simulink model "MEEN432_Project3_Wk3_Model"  (R2024b)
settings: Solver=VariableStepAuto  StartTime=0.0  StopTime=344  RelTol=1e-3
values from neighbouring files (symbols this model uses):
  epa = urban_epa    [Project3_run.m]
  time = urban_time    [Project3_run.m]
undefined symbols (not defined in the file or in its folder): datBat, datCar, datMotor, F_drag, I_w, m, r
libraries: slpidlib x2
settings Model: Creator=flare  LastModifiedBy=jpalm
settings RTWCC: GPUComputeCapability=3.5

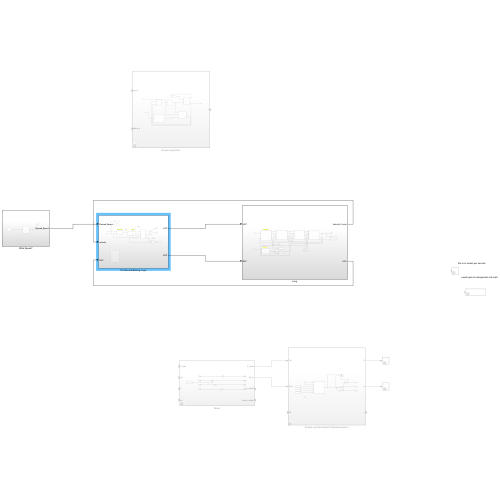
[thumbnail: Simulink's stored preview of the top-level diagram]
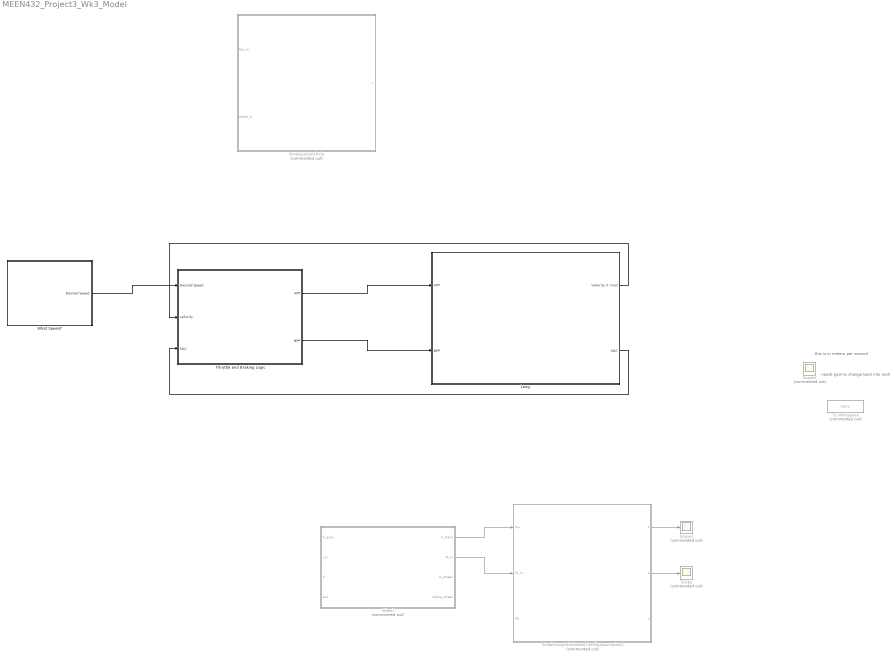
== system MEEN432_Project3_Wk3_Model ==
  note: needs gain to change back into mph
  note: this is in meters per second
  Long. : Subsystem
  Scope : Scope  Commented=on
  Scope1 : Scope  Commented=on
  Scope2 : Scope  Commented=on
  SimpleLongVehicle : Subsystem  Commented=on
  SimpleLongVehiclewNoTireSlipAssumption1 : Subsystem  Commented=on
  Throttle and Braking Logic : Subsystem
  To Workspace : ToWorkspace  Commented=on  VariableName=simv  SaveFormat=Timeseries  SampleTime=-1
  What Speed? : Subsystem
  Wheel : Subsystem  Commented=on
  wires:
  SimpleLongVehiclewNoTireSlipAssumption1/2(a) -> Scope/1
  SimpleLongVehiclewNoTireSlipAssumption1/1(X) -> Scope1/1
  Wheel/1(F_track) -> SimpleLongVehiclewNoTireSlipAssumption1/1(Fw)
  Wheel/2(M_in) -> SimpleLongVehiclewNoTireSlipAssumption1/2(M_in)
  What Speed?/1(Desired Speed) -> Throttle and Braking Logic/1(Desired Speed)
  Throttle and Braking Logic/1(APP) -> Long./1(APP)
  Throttle and Braking Logic/2(BPP) -> Long./2(BPP)
  Long./1(Velocity X (m/s)) -> Throttle and Braking Logic/2(velocity)
  Long./2(SOC) -> Throttle and Braking Logic/3(SOC)

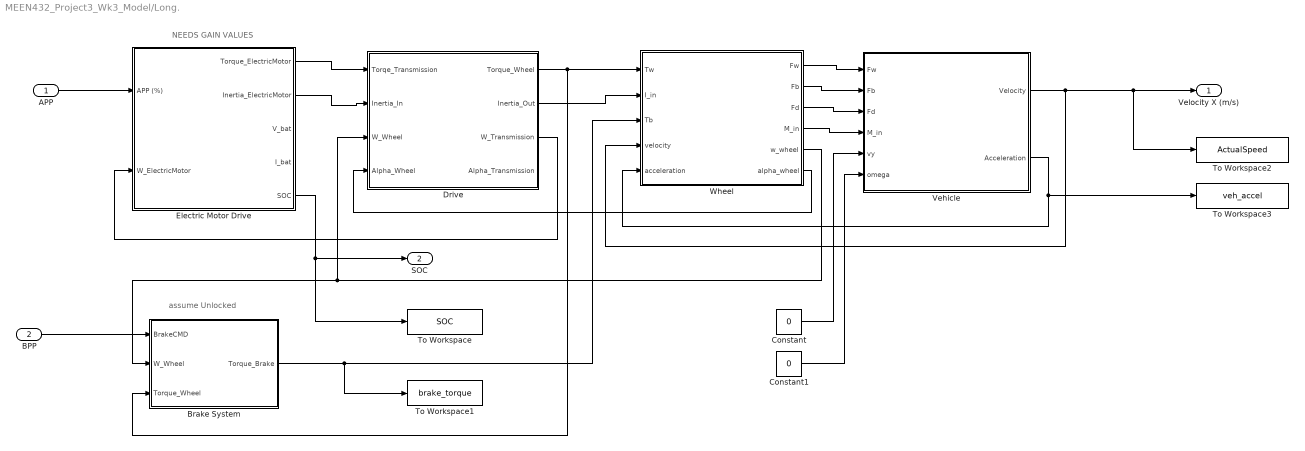
== system MEEN432_Project3_Wk3_Model/Long. ==
  note: assume Unlocked
  note: NEEDS GAIN VALUES
  APP : Inport
  BPP : Inport  Port=2
  Brake System : Subsystem
  Constant : Constant  Value=0
  Constant1 : Constant  Value=0
  Drive : Subsystem
  Electric Motor Drive : Subsystem
  To Workspace : ToWorkspace  VariableName=SOC  SaveFormat=Timeseries  SampleTime=-1
  To Workspace1 : ToWorkspace  VariableName=brake_torque  SaveFormat=Timeseries  SampleTime=-1
  To Workspace2 : ToWorkspace  VariableName=ActualSpeed  SaveFormat=Timeseries  SampleTime=-1
  To Workspace3 : ToWorkspace  VariableName=veh_accel  SaveFormat=Timeseries  SampleTime=-1
  Vehicle : Subsystem
  Wheel : Subsystem
  Velocity X (m/s) : Outport
  SOC : Outport  Port=2
  wires:
  Drive/1(Torque_Wheel) -> Brake System/3(Torque_Wheel), Wheel/1(Tw)
  Drive/2(Inertia_Out) -> Wheel/2(I_in)
  Drive/3(W_Transmission) -> Electric Motor Drive/2(W_ElectricMotor)
  Electric Motor Drive/2(Inertia_ElectricMotor) -> Drive/2(Inertia_In)
  APP/1 -> Electric Motor Drive/1(APP (%))
  BPP/1 -> Brake System/1(BrakeCMD)
  Wheel/5(w_wheel) -> Drive/3(W_Wheel), Brake System/2(W_Wheel)
  Brake System/1(Torque_Brake) -> To Workspace1/1, Wheel/3(Tb)
  Vehicle/1(Velocity) -> Wheel/4(velocity), To Workspace2/1, Velocity X (m/s)/1
  Vehicle/2(Acceleration) -> To Workspace3/1, Wheel/5(acceleration)
  Wheel/1(Fw) -> Vehicle/1(Fw)
  Wheel/2(Fb) -> Vehicle/2(Fb)
  Wheel/3(Fd) -> Vehicle/3(Fd)
  Wheel/4(M_in) -> Vehicle/4(M_in)
  Wheel/6(alpha_wheel) -> Drive/4(Alpha_Wheel)
  Electric Motor Drive/5(SOC) -> To Workspace/1, SOC/1
  Constant/1 -> Vehicle/5(vy)
  Constant1/1 -> Vehicle/6(omega)
  Electric Motor Drive/1(Torque_ElectricMotor) -> Drive/1(Torqe_Transmission)

== system MEEN432_Project3_Wk3_Model/SimpleLongVehicle ==
  note: Is this the torque that we control?
  note: assuming no tire slip for Week 1
  note: still need to saturate
  note: Do we need "Road" and "Brakes" for Wk 1?
  tau_w : Inport
  alpha_b : Inport  Port=2
  Braking : Subsystem
  Long Vehicle Dynamics : Subsystem
  Road : Subsystem
  Tire Longitudinal Force : Subsystem
  Tire Slip Ratio : Subsystem
  Wheel Dynamics : Subsystem
  v : Outport
  wires:
  tau_w/1 -> Wheel Dynamics/2(tau_w)
  Tire Slip Ratio/1(lambda) -> Tire Longitudinal Force/1(lambda)
  alpha_b/1 -> Braking/1(alpha_b)
  Tire Longitudinal Force/1(Fx) -> Long Vehicle Dynamics/2(Fx), Wheel Dynamics/1(Fx)
  Road/1(Theta) -> Long Vehicle Dynamics/1(theta)
  Long Vehicle Dynamics/1(X) -> Road/1(X)
  Braking/1(tau_b) -> Wheel Dynamics/3(tau_b)
  Wheel Dynamics/2(omega_w) -> Tire Slip Ratio/2(omega_w)
  Long Vehicle Dynamics/3(v) -> Tire Slip Ratio/1(v), v/1

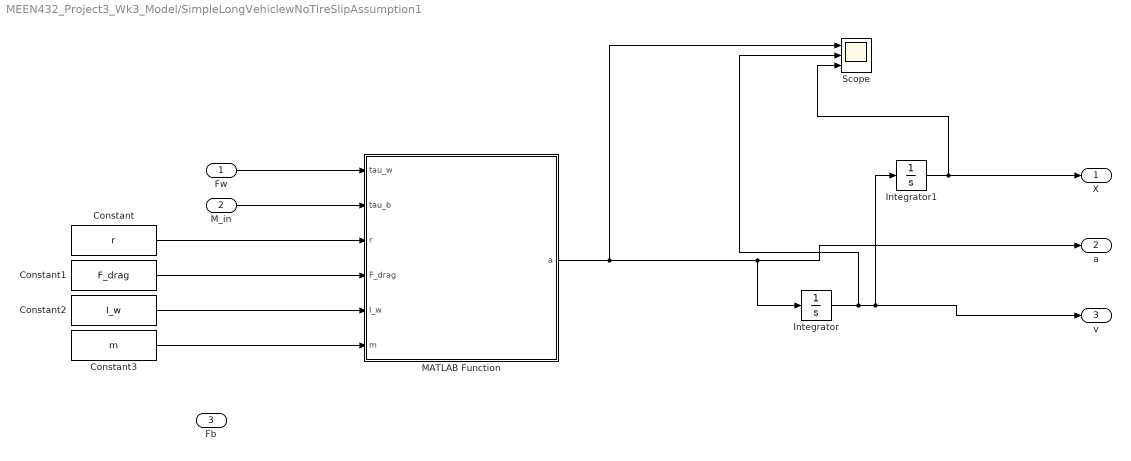
== system MEEN432_Project3_Wk3_Model/SimpleLongVehiclewNoTireSlipAssumption1 ==
  Fw : Inport
  M_in : Inport  Port=2
  Fb : Inport  Port=3
  Constant : Constant  Value=r
  Constant1 : Constant  Value=F_drag
  Constant2 : Constant  Value=I_w
  Constant3 : Constant  Value=m
  Integrator : Integrator
  Integrator1 : Integrator
  MATLAB Function : MATLAB Function  TreatAsAtomicUnit=on
  Scope : Scope  NumInputPorts=3
  X : Outport
  a : Outport  Port=2
  v : Outport  Port=3
  wires:
  MATLAB Function/1(a) -> Scope/1, Integrator/1, a/1
  Integrator/1 -> Scope/2, Integrator1/1, v/1
  Integrator1/1 -> Scope/3, X/1
  Fw/1 -> MATLAB Function/1(tau_w)
  M_in/1 -> MATLAB Function/2(tau_b)
  Constant/1 -> MATLAB Function/3(r)
  Constant1/1 -> MATLAB Function/4(F_drag)
  Constant2/1 -> MATLAB Function/5(I_w)
  Constant3/1 -> MATLAB Function/6(m)

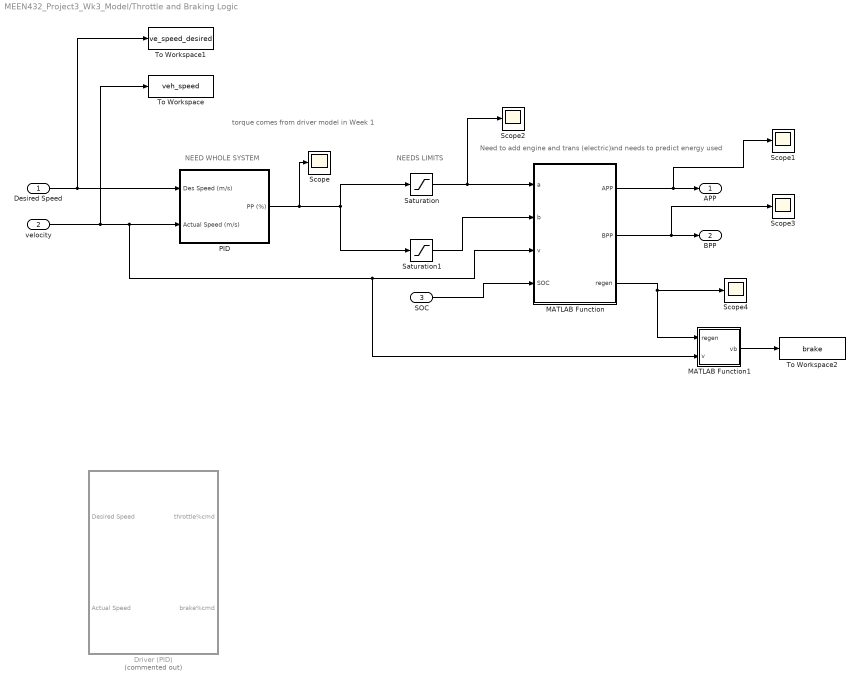
== system MEEN432_Project3_Wk3_Model/Throttle and Braking Logic ==
  note: NEEDS LIMITS
  note: NEED WHOLE SYSTEM
  note: and needs to predict energy used
  note: Need to add engine and trans (electric)
  note: torque comes from driver model in Week 1
  Desired Speed : Inport
  velocity : Inport  Port=2
  SOC : Inport  Port=3
  Driver (PID) : Subsystem  Commented=on
  MATLAB Function : MATLAB Function  TreatAsAtomicUnit=on
  MATLAB Function1 : MATLAB Function  TreatAsAtomicUnit=on
  PID : Subsystem
  Saturation : Saturate  UpperLimit=1  LowerLimit=0
  Saturation1 : Saturate  UpperLimit=0  LowerLimit=-1
  Scope{,1..4} (5 alike) : Scope
  To Workspace : ToWorkspace  VariableName=veh_speed  SaveFormat=Timeseries  SampleTime=-1
  To Workspace1 : ToWorkspace  VariableName=ve_speed_desired  SaveFormat=Timeseries  SampleTime=-1
  To Workspace2 : ToWorkspace  VariableName=brake  SaveFormat=Timeseries  SampleTime=-1
  APP : Outport
  BPP : Outport  Port=2
  wires:
  Desired Speed/1 -> PID/1(Des Speed (m/s)), To Workspace1/1
  velocity/1 -> To Workspace/1, MATLAB Function1/2(v), MATLAB Function/3(v), PID/2(Actual Speed (m/s))
  PID/1(PP (%)) -> Scope/1, Saturation1/1, Saturation/1
  Saturation1/1 -> MATLAB Function/2(b)
  Saturation/1 -> Scope2/1, MATLAB Function/1(a)
  SOC/1 -> MATLAB Function/4(SOC)
  MATLAB Function/3(regen) -> MATLAB Function1/1(regen), Scope4/1
  MATLAB Function1/1(vb) -> To Workspace2/1
  MATLAB Function/2(BPP) -> Scope3/1, BPP/1
  MATLAB Function/1(APP) -> Scope1/1, APP/1

== system MEEN432_Project3_Wk3_Model/What Speed? ==
  1-D Lookup Table : Lookup_n-D  NumberOfTableDimensions=1  BreakpointsForDimension1=time  Table=epa  InternalRulePriority=Speed  RndMeth=Simplest
  Clock : Clock
  Scope : Scope
  mph to mps : Gain  Gain=0.44704
  Desired Speed : Outport
  wires:
  Clock/1 -> 1-D Lookup Table/1
  1-D Lookup Table/1 -> mph to mps/1
  mph to mps/1 -> Scope/1, Desired Speed/1

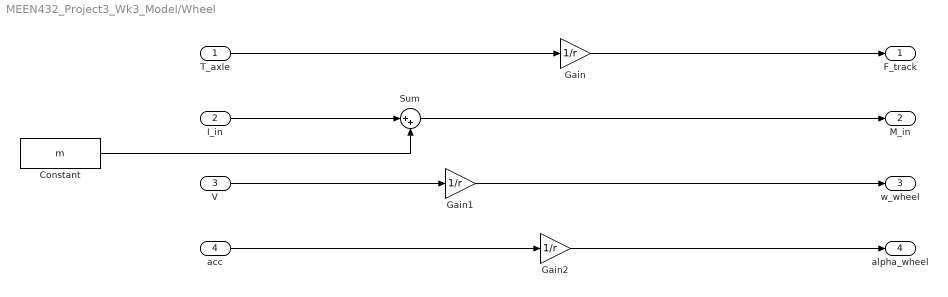
== system MEEN432_Project3_Wk3_Model/Wheel ==
  T_axle : Inport
  I_in : Inport  Port=2
  V : Inport  Port=3
  acc : Inport  Port=4
  Constant : Constant  Value=m
  Gain : Gain  Gain=1/r
  Gain1 : Gain  Gain=1/r
  Gain2 : Gain  Gain=1/r
  Sum : Sum  Inputs=|++
  F_track : Outport
  M_in : Outport  Port=2
  w_wheel : Outport  Port=3
  alpha_wheel : Outport  Port=4
  wires:
  T_axle/1 -> Gain/1
  Gain/1 -> F_track/1
  I_in/1 -> Sum/1
  Sum/1 -> M_in/1
  Constant/1 -> Sum/2
  V/1 -> Gain1/1
  Gain1/1 -> w_wheel/1
  acc/1 -> Gain2/1
  Gain2/1 -> alpha_wheel/1

== system MEEN432_Project3_Wk3_Model/Long./Brake System ==
  BrakeCMD : Inport
  W_Wheel : Inport  Port=2
  Torque_Wheel : Inport  Port=3
  Constant : Constant  Value=datCar.maxBrakeTorque
  Constant1 : Constant  Value=datCar.brakeGeometricDesign
  Constant2 : Constant  Value=datCar.brakeFriction
  MATLAB Function : MATLAB Function  TreatAsAtomicUnit=on
  Scope : Scope
  Torque_Brake : Outport
  wires:
  BrakeCMD/1 -> MATLAB Function/1(alpha_b)
  W_Wheel/1 -> MATLAB Function/5(omega_w)
  MATLAB Function/1(tau_b) -> Scope/1, Torque_Brake/1
  Constant/1 -> MATLAB Function/3(N_b_max)
  Constant1/1 -> MATLAB Function/4(g_b)
  Constant2/1 -> MATLAB Function/2(mu_b)

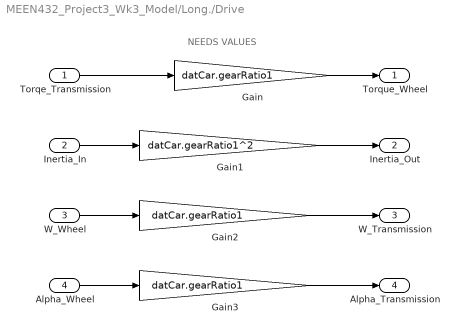
== system MEEN432_Project3_Wk3_Model/Long./Drive ==
  note: NEEDS VALUES
  Torqe_Transmission : Inport
  Inertia_In : Inport  Port=2
  W_Wheel : Inport  Port=3
  Alpha_Wheel : Inport  Port=4
  Gain : Gain  Gain=datCar.gearRatio1
  Gain1 : Gain  Gain=datCar.gearRatio1^2
  Gain2 : Gain  Gain=datCar.gearRatio1
  Gain3 : Gain  Gain=datCar.gearRatio1
  Torque_Wheel : Outport
  Inertia_Out : Outport  Port=2
  W_Transmission : Outport  Port=3
  Alpha_Transmission : Outport  Port=4
  wires:
  Torqe_Transmission/1 -> Gain/1
  Inertia_In/1 -> Gain1/1
  W_Wheel/1 -> Gain2/1
  Alpha_Wheel/1 -> Gain3/1
  Gain3/1 -> Alpha_Transmission/1
  Gain2/1 -> W_Transmission/1
  Gain1/1 -> Inertia_Out/1
  Gain/1 -> Torque_Wheel/1

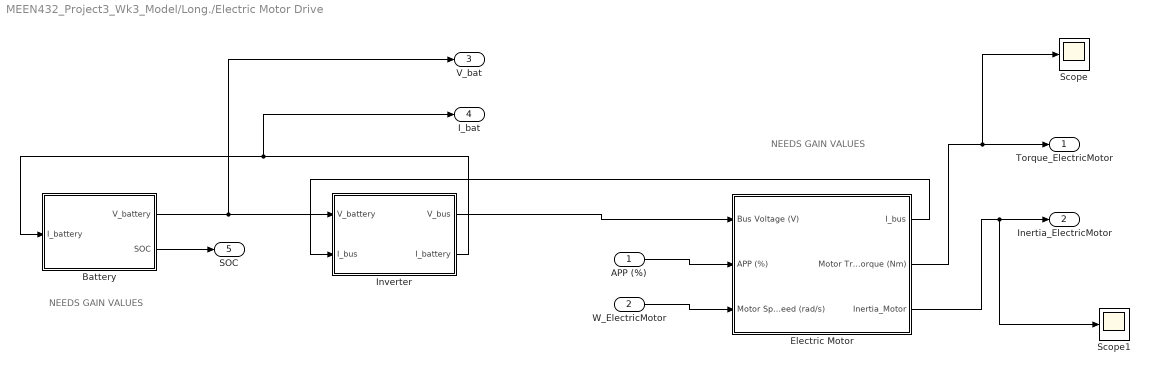
== system MEEN432_Project3_Wk3_Model/Long./Electric Motor Drive ==
  note: NEEDS GAIN VALUES
  note: NEEDS GAIN VALUES
  APP (%) : Inport
  W_ElectricMotor : Inport  Port=2
  Battery : Subsystem
  Electric Motor : Subsystem
  Inverter : Subsystem
  Scope : Scope
  Scope1 : Scope
  Torque_ElectricMotor : Outport
  Inertia_ElectricMotor : Outport  Port=2
  V_bat : Outport  Port=3
  I_bat : Outport  Port=4
  SOC : Outport  Port=5
  wires:
  APP (%)/1 -> Electric Motor/2(APP (%))
  W_ElectricMotor/1 -> Electric Motor/3(Motor Speed (rad/s))
  Inverter/1(V_bus) -> Electric Motor/1(Bus Voltage (V))
  Battery/1(V_battery) -> V_bat/1, Inverter/1(V_battery)
  Inverter/2(I_battery) -> I_bat/1, Battery/1(I_battery)
  Electric Motor/1(I_bus) -> Inverter/2(I_bus)
  Electric Motor/2(Motor Trorque (Nm)) -> Scope/1, Torque_ElectricMotor/1
  Electric Motor/3(Inertia_Motor) -> Scope1/1, Inertia_ElectricMotor/1
  Battery/2(SOC) -> SOC/1

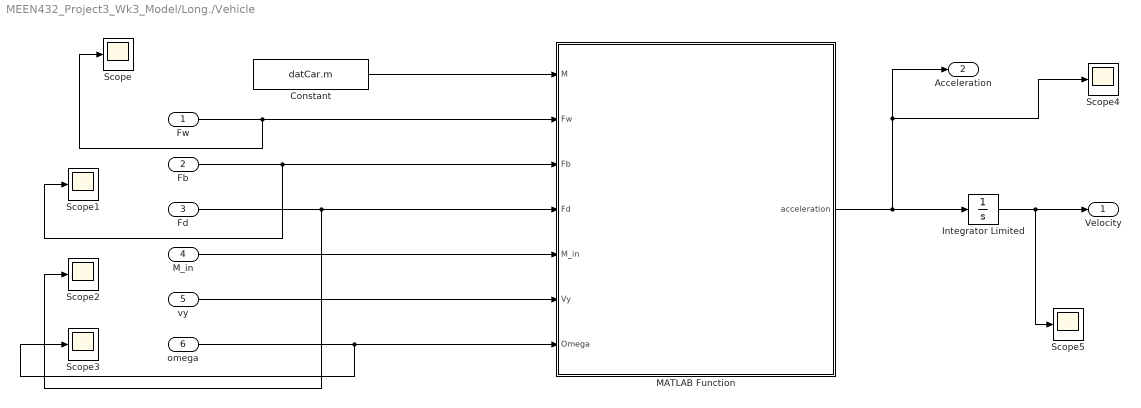
== system MEEN432_Project3_Wk3_Model/Long./Vehicle ==
  Fw : Inport
  Fb : Inport  Port=2
  Fd : Inport  Port=3
  M_in : Inport  Port=4
  vy : Inport  Port=5
  omega : Inport  Port=6
  Constant : Constant  Value=datCar.m
  Integrator Limited : Integrator  LimitOutput=on  UpperSaturationLimit=10000  LowerSaturationLimit=0
  MATLAB Function : MATLAB Function  TreatAsAtomicUnit=on
  Scope{,1..5} (6 alike) : Scope
  Velocity : Outport
  Acceleration : Outport  Port=2
  wires:
  omega/1 -> Scope3/1, MATLAB Function/7(Omega)
  vy/1 -> MATLAB Function/6(Vy)
  M_in/1 -> MATLAB Function/5(M_in)
  Fb/1 -> Scope1/1, MATLAB Function/3(Fb)
  Fw/1 -> Scope/1, MATLAB Function/2(Fw)
  MATLAB Function/1(acceleration) -> Integrator Limited/1, Scope4/1, Acceleration/1
  Integrator Limited/1 -> Scope5/1, Velocity/1
  Constant/1 -> MATLAB Function/1(M)
  Fd/1 -> Scope2/1, MATLAB Function/4(Fd)

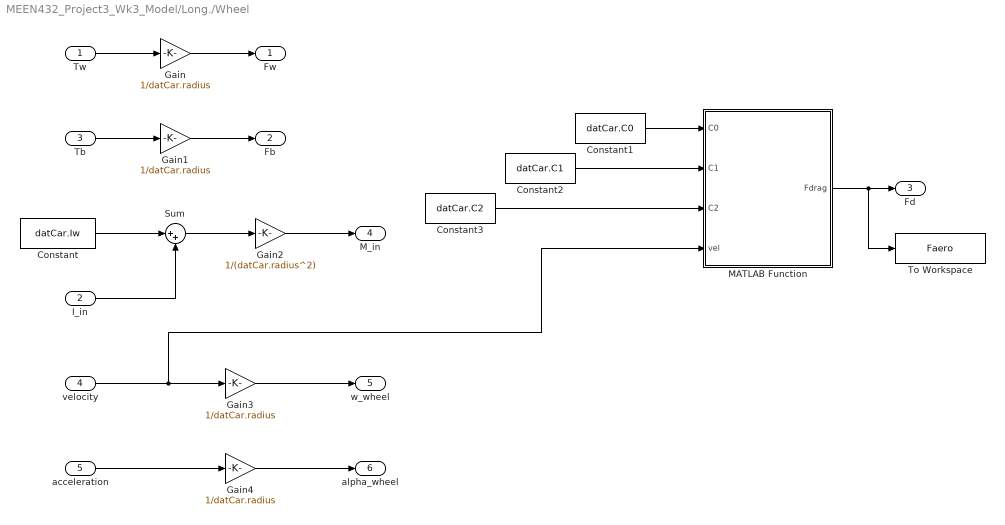
== system MEEN432_Project3_Wk3_Model/Long./Wheel ==
  Tw : Inport
  I_in : Inport  Port=2
  Tb : Inport  Port=3
  velocity : Inport  Port=4
  acceleration : Inport  Port=5
  Constant : Constant  Value=datCar.Iw
  Constant1 : Constant  Value=datCar.C0
  Constant2 : Constant  Value=datCar.C1
  Constant3 : Constant  Value=datCar.C2
  Gain{,1,3..4} (4 alike) : Gain  Gain=1/datCar.radius
  Gain2 : Gain  Gain=1/(datCar.radius^2)
  MATLAB Function : MATLAB Function  TreatAsAtomicUnit=on
  Sum : Sum  Inputs=|++
  To Workspace : ToWorkspace  VariableName=Faero  SaveFormat=Timeseries  SampleTime=-1
  Fw : Outport
  Fb : Outport  Port=2
  Fd : Outport  Port=3
  M_in : Outport  Port=4
  w_wheel : Outport  Port=5
  alpha_wheel : Outport  Port=6
  wires:
  Tw/1 -> Gain/1
  Gain/1 -> Fw/1
  Gain1/1 -> Fb/1
  Tb/1 -> Gain1/1
  Constant/1 -> Sum/1
  I_in/1 -> Sum/2
  Sum/1 -> Gain2/1
  Gain2/1 -> M_in/1
  velocity/1 -> MATLAB Function/4(vel), Gain3/1
  acceleration/1 -> Gain4/1
  Gain3/1 -> w_wheel/1
  Gain4/1 -> alpha_wheel/1
  MATLAB Function/1(Fdrag) -> To Workspace/1, Fd/1
  Constant1/1 -> MATLAB Function/1(C0)
  Constant2/1 -> MATLAB Function/2(C1)
  Constant3/1 -> MATLAB Function/3(C2)

== system MEEN432_Project3_Wk3_Model/SimpleLongVehicle/Braking ==
  note: assuming only locked?
  alpha_b : Inport
  Braking : MATLAB Function  TreatAsAtomicUnit=on
  Constant{,1..3} (4 alike) : Constant
  tau_b : Outport
  wires:
  Braking/1(tau_b) -> tau_b/1
  alpha_b/1 -> Braking/1(alpha_b)
  Constant/1 -> Braking/2(mu_b)
  Constant1/1 -> Braking/3(N_b_max)
  Constant2/1 -> Braking/5(omega_w)
  Constant3/1 -> Braking/4(g_b)

== system MEEN432_Project3_Wk3_Model/SimpleLongVehicle/Long Vehicle Dynamics ==
  theta : Inport
  Fx : Inport  Port=2
  Constant : Constant
  Constant1 : Constant
  Long Vehicle Dynamics : MATLAB Function  TreatAsAtomicUnit=on
  X : Outport
  a : Outport  Port=2
  v : Outport  Port=3
  wires:
  theta/1 -> Long Vehicle Dynamics/1(theta)
  Long Vehicle Dynamics/1(omega_dot) -> a/1
  Fx/1 -> Long Vehicle Dynamics/2(Fx)
  Constant/1 -> Long Vehicle Dynamics/3(r)
  Constant1/1 -> Long Vehicle Dynamics/4(F_drag)

== system MEEN432_Project3_Wk3_Model/SimpleLongVehicle/Road ==
  X : Inport
  Theta : Outport
  wires:
  X/1 -> Theta/1

== system MEEN432_Project3_Wk3_Model/SimpleLongVehicle/Tire Longitudinal Force ==
  lambda : Inport
  Tire Longitudinal Force : MATLAB Function  TreatAsAtomicUnit=on
  Fx : Outport
  wires:
  lambda/1 -> Tire Longitudinal Force/1(lambda)
  Tire Longitudinal Force/1(Fx) -> Fx/1

== system MEEN432_Project3_Wk3_Model/SimpleLongVehicle/Tire Slip Ratio ==
  v : Inport
  omega_w : Inport  Port=2
  Tire Slip Ratio : MATLAB Function  TreatAsAtomicUnit=on
  Wheel Radius : Constant
  lambda : Outport
  wires:
  v/1 -> Tire Slip Ratio/1(v)
  Tire Slip Ratio/1(lambda) -> lambda/1
  omega_w/1 -> Tire Slip Ratio/3(omega_w)
  Wheel Radius/1 -> Tire Slip Ratio/2(r_w)

== system MEEN432_Project3_Wk3_Model/SimpleLongVehicle/Wheel Dynamics ==
  Fx : Inport
  tau_w : Inport  Port=2
  tau_b : Inport  Port=3
  Constant : Constant
  Constant1 : Constant
  Integrator : Integrator
  Wheel Dynamics : MATLAB Function  TreatAsAtomicUnit=on
  omega_w_dot : Outport
  omega_w : Outport  Port=2
  wires:
  Fx/1 -> Wheel Dynamics/1(Fx)
  tau_w/1 -> Wheel Dynamics/2(tau_w)
  tau_b/1 -> Wheel Dynamics/3(tau_b)
  Wheel Dynamics/1(omega_w_dot) -> Integrator/1, omega_w_dot/1
  Constant/1 -> Wheel Dynamics/4(r_w)
  Constant1/1 -> Wheel Dynamics/5(I)
  Integrator/1 -> omega_w/1

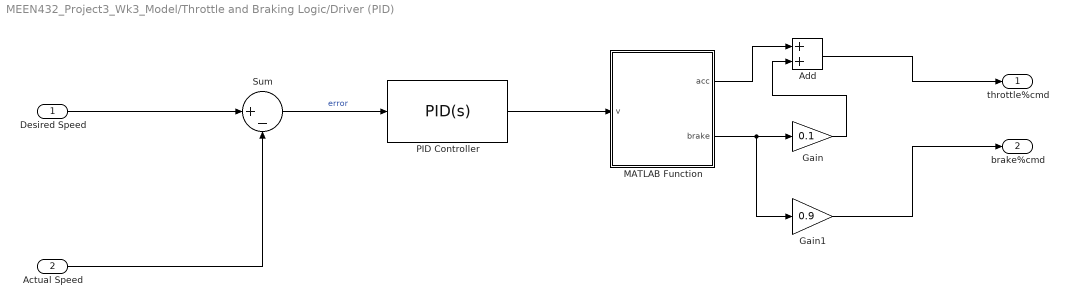
== system MEEN432_Project3_Wk3_Model/Throttle and Braking Logic/Driver (PID) ==
  Desired Speed : Inport
  Actual Speed : Inport  Port=2
  Add : Sum
  Gain : Gain  Gain=0.1
  Gain1 : Gain  Gain=0.9
  MATLAB Function : MATLAB Function  TreatAsAtomicUnit=on
  PID Controller : slpidlib/PID Controller  Controller=PID  Form=Parallel  TimeDomain=Continuous-time  UseExternalTs=off  SampleTime=-1  IntegratorMethod=Forward Euler  FilterMethod=Forward Euler  ControllerParametersSource=internal  P=1  I=1  UseKiTs=off  D=0  UseExternalDerivativeSource=off  N=100  UseFilter=on  TunerSelectOption=Transfer Function Based (PID Tuner App)  InitialConditionSource=internal  InitialConditionForIntegrator=0  InitialConditionForFilter=0  DifferentiatorICPrevScaledInput=0  ExternalReset=none  TrackingMode=off  Kt=1  LimitOutput=off  SatLimitsSource=internal  UpperSaturationLimit=inf  LowerSaturationLimit=-inf  LinearizeAsGain=on  AntiWindupMode=none  Kb=1  LimitIntegrator=off  UpperIntegratorSaturationLimit=inf  LowerIntegratorSaturationLimit=-inf  POutMin=[]  POutMax=[]  IOutMin=[]  IOutMax=[]  DOutMin=[]  DOutMax=[]  NOutMin=[]  NOutMax=[]  SumOutMin=[]  SumOutMax=[]  SaturationOutMin=[]  SaturationOutMax=[]  PParamMin=[]  PParamMax=[]  IParamMin=[]  IParamMax=[]  DParamMin=[]  DParamMax=[]  NParamMin=[]  NParamMax=[]  KbParamMin=[]  KbParamMax=[]  KtParamMin=[]  KtParamMax=[]  KbOutMin=[]  KbOutMax=[]  KtOutMin=[]  KtOutMax=[]  IntegratorOutMin=[]  IntegratorOutMax=[]  FilterOutMin=[]  FilterOutMax=[]  SumI1OutMin=[]  SumI1OutMax=[]  SumI2OutMin=[]  SumI2OutMax=[]  SumI3OutMin=[]  SumI3OutMax=[]  SumI4OutMin=[]  SumI4OutMax=[]  SumDOutMin=[]  SumDOutMax=[]  DifferentiatorOutMin=[]  DifferentiatorOutMax=[]  FilterDiffOutCoefMin=[]  FilterDiffOutCoefMax=[]  ReciprocalOutMin=[]  ReciprocalOutMax=[]  SumDenOutMin=[]  SumDenOutMax=[]  SumNumOutMin=[]  SumNumOutMax=[]  DivideOutMin=[]  DivideOutMax=[]  UdiffTsProdOutMin=[]  UdiffTsProdOutMax=[]  NTsProdOutMin=[]  NTsProdOutMax=[]  UintegralTsProdOutMin=[]  UintegralTsProdOutMax=[]  UngainTsProdOutMin=[]  UngainTsProdOutMax=[]  ClampingZeroOutDataTypeStr=Inherit: Inherit via back propagation  ClampingZeroOutMin=[]  ClampingZeroOutMax=[]  FilterDenConstantOutDataTypeStr=Inherit: Inherit via back propagation  FilterDenConstantOutMin=[]  FilterDenConstantOutMax=[]  PCopyOutDataTypeStr=Inherit: Inherit via back propagation  PCopyOutMin=[]  PCopyOutMax=[]  NCopyOutDataTypeStr=Inherit: Inherit via back propagation  NCopyOutMin=[]  NCopyOutMax=[]  IntegratorContinuousStateAttributes=''  IntegratorStateMustResolveToSignalObject=off  IntegratorRTWStateStorageClass=Auto  FilterContinuousStateAttributes=''  FilterStateMustResolveToSignalObject=off  FilterRTWStateStorageClass=Auto  ParallelPVariant=InternalParameters  IdealPVariant=Disabled  IVariant=InternalParameters  DVariant=InternalParameters  IntegratorVariant=Continuous  SatVariant=Disabled  AWVariant=Passthrough  PCopyVariant=Disabled  TRVariant=Disabled  FdbkBlocksVariant=Forward  IdealPFdbkVariant=Disabled  SatFdbkVariant=Disabled  DerivativeFilterVariant=ContFilter  NVariant=InternalParameters  NCopyVariant=Disabled  FilterICVariant=InternalICsFilter  IntegratorICVariant=InternalICs  ExternalResetVariant=Disabled  TRSumVariant=Passthrough  SumFdbkVariant=Disabled  SumVariant=Sum_PID  TsampFilterVariant=InternalTs  TsampNgainVariant=Passthrough  TsampIntegralVariant=Disabled_SignalSpec  ExternalSaturationOutDataTypeStr=Inherit: Same as second input  DerivativeSourceVariant=ErrorSignal  PreIntVariant=InternalPreInt
  Sum : Sum  Inputs=|+-
  throttle%cmd : Outport
  brake%cmd : Outport  Port=2
  wires:
  Actual Speed/1 -> Sum/2
  Sum/1 -> PID Controller/1  "error"
  PID Controller/1 -> MATLAB Function/1(v)
  MATLAB Function/1(acc) -> Add/1
  MATLAB Function/2(brake) -> Gain1/1, Gain/1
  Gain/1 -> Add/2
  Gain1/1 -> brake%cmd/1
  Add/1 -> throttle%cmd/1
  Desired Speed/1 -> Sum/1

== system MEEN432_Project3_Wk3_Model/Throttle and Braking Logic/PID ==
  Des Speed (m/s) : Inport
  Actual Speed (m/s) : Inport  Port=2
  PID Controller : slpidlib/PID Controller  Controller=PID  Form=Parallel  TimeDomain=Continuous-time  UseExternalTs=off  SampleTime=-1  IntegratorMethod=Forward Euler  FilterMethod=Forward Euler  ControllerParametersSource=internal  P=1000  I=1  UseKiTs=off  D=0  UseExternalDerivativeSource=off  N=100  UseFilter=on  TunerSelectOption=Transfer Function Based (PID Tuner App)  InitialConditionSource=internal  InitialConditionForIntegrator=0  InitialConditionForFilter=0  DifferentiatorICPrevScaledInput=0  ExternalReset=none  TrackingMode=off  Kt=1  LimitOutput=off  SatLimitsSource=internal  UpperSaturationLimit=inf  LowerSaturationLimit=-inf  LinearizeAsGain=on  AntiWindupMode=none  Kb=1  LimitIntegrator=off  UpperIntegratorSaturationLimit=inf  LowerIntegratorSaturationLimit=-inf  POutMin=[]  POutMax=[]  IOutMin=[]  IOutMax=[]  DOutMin=[]  DOutMax=[]  NOutMin=[]  NOutMax=[]  SumOutMin=[]  SumOutMax=[]  SaturationOutMin=[]  SaturationOutMax=[]  PParamMin=[]  PParamMax=[]  IParamMin=[]  IParamMax=[]  DParamMin=[]  DParamMax=[]  NParamMin=[]  NParamMax=[]  KbParamMin=[]  KbParamMax=[]  KtParamMin=[]  KtParamMax=[]  KbOutMin=[]  KbOutMax=[]  KtOutMin=[]  KtOutMax=[]  IntegratorOutMin=[]  IntegratorOutMax=[]  FilterOutMin=[]  FilterOutMax=[]  SumI1OutMin=[]  SumI1OutMax=[]  SumI2OutMin=[]  SumI2OutMax=[]  SumI3OutMin=[]  SumI3OutMax=[]  SumI4OutMin=[]  SumI4OutMax=[]  SumDOutMin=[]  SumDOutMax=[]  DifferentiatorOutMin=[]  DifferentiatorOutMax=[]  FilterDiffOutCoefMin=[]  FilterDiffOutCoefMax=[]  ReciprocalOutMin=[]  ReciprocalOutMax=[]  SumDenOutMin=[]  SumDenOutMax=[]  SumNumOutMin=[]  SumNumOutMax=[]  DivideOutMin=[]  DivideOutMax=[]  UdiffTsProdOutMin=[]  UdiffTsProdOutMax=[]  NTsProdOutMin=[]  NTsProdOutMax=[]  UintegralTsProdOutMin=[]  UintegralTsProdOutMax=[]  UngainTsProdOutMin=[]  UngainTsProdOutMax=[]  ClampingZeroOutDataTypeStr=Inherit: Inherit via back propagation  ClampingZeroOutMin=[]  ClampingZeroOutMax=[]  FilterDenConstantOutDataTypeStr=Inherit: Inherit via back propagation  FilterDenConstantOutMin=[]  FilterDenConstantOutMax=[]  PCopyOutDataTypeStr=Inherit: Inherit via back propagation  PCopyOutMin=[]  PCopyOutMax=[]  NCopyOutDataTypeStr=Inherit: Inherit via back propagation  NCopyOutMin=[]  NCopyOutMax=[]  IntegratorContinuousStateAttributes=''  IntegratorStateMustResolveToSignalObject=off  IntegratorRTWStateStorageClass=Auto  FilterContinuousStateAttributes=''  FilterStateMustResolveToSignalObject=off  FilterRTWStateStorageClass=Auto  ParallelPVariant=InternalParameters  IdealPVariant=Disabled  IVariant=InternalParameters  DVariant=InternalParameters  IntegratorVariant=Continuous  SatVariant=Disabled  AWVariant=Passthrough  PCopyVariant=Disabled  TRVariant=Disabled  FdbkBlocksVariant=Forward  IdealPFdbkVariant=Disabled  SatFdbkVariant=Disabled  DerivativeFilterVariant=ContFilter  NVariant=InternalParameters  NCopyVariant=Disabled  FilterICVariant=InternalICsFilter  IntegratorICVariant=InternalICs  ExternalResetVariant=Disabled  TRSumVariant=Passthrough  SumFdbkVariant=Disabled  SumVariant=Sum_PID  TsampFilterVariant=InternalTs  TsampNgainVariant=Passthrough  TsampIntegralVariant=Disabled_SignalSpec  ExternalSaturationOutDataTypeStr=Inherit: Same as second input  DerivativeSourceVariant=ErrorSignal  PreIntVariant=InternalPreInt
  Saturation : Saturate  UpperLimit=1  LowerLimit=-1
  Scope{,1..3} (4 alike) : Scope
  Sum : Sum  Inputs=|+-
  PP (%) : Outport
  wires:
  Sum/1 -> Scope/1, PID Controller/1
  PID Controller/1 -> Saturation/1, Scope2/1
  Des Speed (m/s)/1 -> Sum/1
  Actual Speed (m/s)/1 -> Scope3/1, Sum/2
  Saturation/1 -> Scope1/1, PP (%)/1

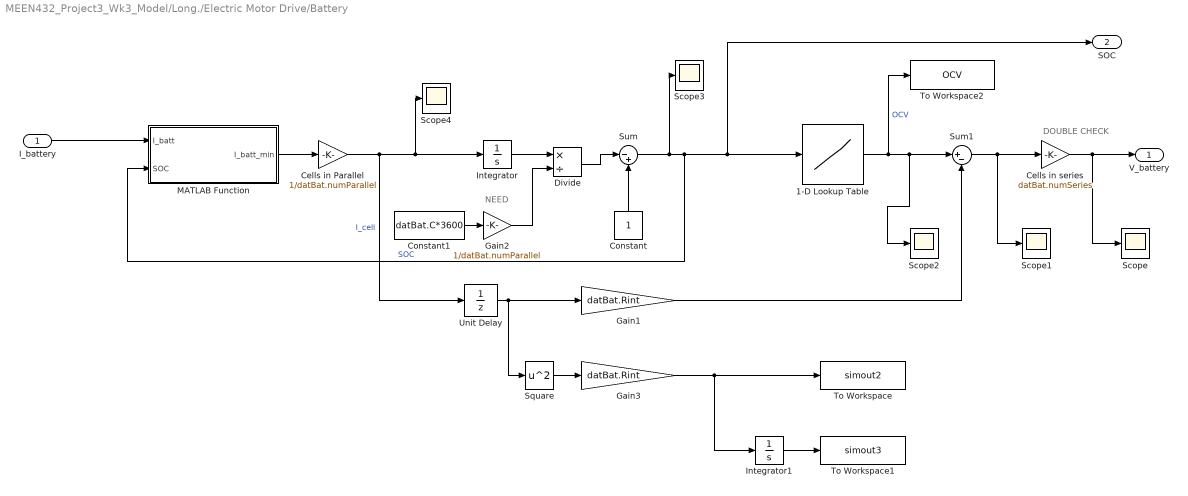
== system MEEN432_Project3_Wk3_Model/Long./Electric Motor Drive/Battery ==
  note: NEED
  note: DOUBLE CHECK
  I_battery : Inport
  1-D Lookup Table : Lookup_n-D  NumberOfTableDimensions=1  BreakpointsForDimension1=datBat.SOC  Table=datBat.OCV  InternalRulePriority=Speed  RndMeth=Simplest
  Cells in Parallel : Gain  Gain=1/datBat.numParallel
  Cells in series : Gain  Gain=datBat.numSeries
  Constant : Constant
  Constant1 : Constant  Value=datBat.C*3600
  Divide : Product  Inputs=*/
  Gain1 : Gain  Gain=datBat.Rint
  Gain2 : Gain  Gain=1/datBat.numParallel
  Gain3 : Gain  Gain=datBat.Rint
  Integrator : Integrator
  Integrator1 : Integrator
  MATLAB Function : MATLAB Function  TreatAsAtomicUnit=on
  Scope{,1..4} (5 alike) : Scope
  Square : Math  Operator=square
  Sum : Sum  Inputs=|-+
  Sum1 : Sum  Inputs=|+-
  To Workspace : ToWorkspace  VariableName=simout2  SaveFormat=Timeseries  SampleTime=-1
  To Workspace1 : ToWorkspace  VariableName=simout3  SaveFormat=Timeseries  SampleTime=-1
  To Workspace2 : ToWorkspace  VariableName=OCV  SaveFormat=Timeseries  SampleTime=-1
  Unit Delay : UnitDelay  SampleTime=-1  HasFrameUpgradeWarning=on
  V_battery : Outport
  SOC : Outport  Port=2
  wires:
  I_battery/1 -> MATLAB Function/1(I_batt)
  Cells in Parallel/1 -> Scope4/1, Integrator/1, Unit Delay/1  "I_cell"
  Unit Delay/1 -> Square/1, Gain1/1
  Constant/1 -> Sum/2
  Sum/1 -> Scope3/1, MATLAB Function/2(SOC), SOC/1, 1-D Lookup Table/1  "SOC"
  Constant1/1 -> Gain2/1
  Gain3/1 -> Integrator1/1, To Workspace/1
  Integrator1/1 -> To Workspace1/1
  Square/1 -> Gain3/1
  1-D Lookup Table/1 -> To Workspace2/1, Scope2/1, Sum1/1  "OCV"
  Gain1/1 -> Sum1/2
  Sum1/1 -> Scope1/1, Cells in series/1
  Cells in series/1 -> Scope/1, V_battery/1
  Integrator/1 -> Divide/1
  Gain2/1 -> Divide/2
  Divide/1 -> Sum/1
  MATLAB Function/1(I_batt_min) -> Cells in Parallel/1

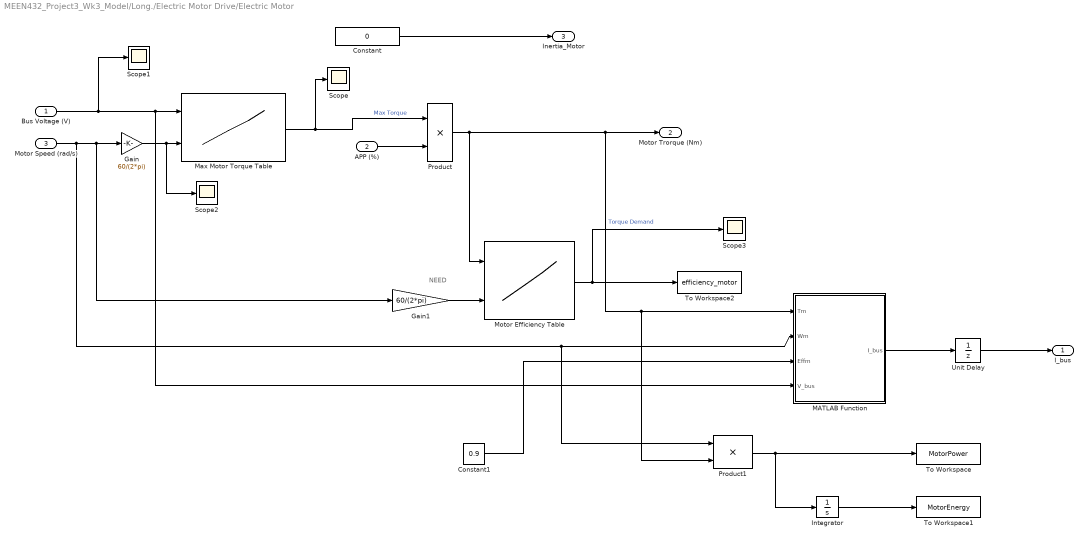
== system MEEN432_Project3_Wk3_Model/Long./Electric Motor Drive/Electric Motor ==
  note: NEED
  Bus Voltage (V) : Inport
  APP (%) : Inport  Port=2
  Motor Speed (rad/s) : Inport  Port=3
  Constant : Constant  Value=0
  Constant1 : Constant  Value=0.9
  Gain : Gain  Gain=60/(2*pi)
  Gain1 : Gain  Gain=60/(2*pi)
  Integrator : Integrator
  MATLAB Function : MATLAB Function  TreatAsAtomicUnit=on
  Max Motor Torque Table : Lookup_n-D  BreakpointsForDimension1=datMotor.vbus  BreakpointsForDimension2=datMotor.rpm  Table=datMotor.maxtorque  InternalRulePriority=Speed  RndMeth=Simplest
      settings: InputPortMap=u0,u1
  Motor Efficiency Table : Lookup_n-D  BreakpointsForDimension1=datMotor.eta_torque  BreakpointsForDimension2=datMotor.eta_speed  Table=datMotor.eta_val  InternalRulePriority=Speed  RndMeth=Simplest
      settings: InputPortMap=u0,u1
  Product : Product
  Product1 : Product
  Scope{,1..3} (4 alike) : Scope
  To Workspace : ToWorkspace  VariableName=MotorPower  SaveFormat=Timeseries  SampleTime=-1
  To Workspace1 : ToWorkspace  VariableName=MotorEnergy  SaveFormat=Timeseries  SampleTime=-1
  To Workspace2 : ToWorkspace  VariableName=efficiency_motor  SaveFormat=Timeseries  SampleTime=-1
  Unit Delay : UnitDelay  SampleTime=-1  HasFrameUpgradeWarning=on
  I_bus : Outport
  Motor Trorque (Nm) : Outport  Port=2
  Inertia_Motor : Outport  Port=3
  wires:
  Bus Voltage (V)/1 -> Scope1/1, MATLAB Function/4(V_bus), Max Motor Torque Table/1
  Motor Speed (rad/s)/1 -> Gain/1, Gain1/1, Product1/1, MATLAB Function/2(Wm)
  Gain/1 -> Scope2/1, Max Motor Torque Table/2
  Max Motor Torque Table/1 -> Scope/1, Product/1  "Max Torque"
  APP (%)/1 -> Product/2
  Constant/1 -> Inertia_Motor/1
  Product/1 -> Product1/2, MATLAB Function/1(Tm), Motor Trorque (Nm)/1, Motor Efficiency Table/1  "Torque Demand"
  Gain1/1 -> Motor Efficiency Table/2
  Motor Efficiency Table/1 -> Scope3/1, To Workspace2/1
  Unit Delay/1 -> I_bus/1
  MATLAB Function/1(I_bus) -> Unit Delay/1
  Product1/1 -> Integrator/1, To Workspace/1
  Integrator/1 -> To Workspace1/1
  Constant1/1 -> MATLAB Function/3(Effm)

== system MEEN432_Project3_Wk3_Model/Long./Electric Motor Drive/Inverter ==
  V_battery : Inport
  I_bus : Inport  Port=2
  Efficiency Inverter : Constant  Value=0.95
  MATLAB Function : MATLAB Function  TreatAsAtomicUnit=on
  Scope : Scope
  Scope1 : Scope
  V_bus : Outport
  I_battery : Outport  Port=2
  wires:
  V_battery/1 -> Scope1/1, MATLAB Function/1(V_bat)
  Efficiency Inverter/1 -> MATLAB Function/2(Eff_I)
  I_bus/1 -> MATLAB Function/3(I_bus)
  MATLAB Function/1(V_bus) -> Scope/1, V_bus/1
  MATLAB Function/2(I_bat) -> I_battery/1

== matlab function MEEN432_Project3_Wk3_Model/Long./Electric Motor Drive/Battery/MATLAB Function ==
  data: I_batt input; I_batt_min output; SOC input
function I_batt_min = fcn(I_batt, SOC)
    if SOC <= 0.1
        I_batt_min = 0;
    else
        I_batt_min = I_batt;
    end

== matlab function MEEN432_Project3_Wk3_Model/Throttle and Braking Logic/MATLAB Function ==
  data: a input; APP output; b input; v input; SOC input; BPP output; regen output
function [APP, BPP, regen] = fcn(a, b, v, SOC)
    if v < (5*(1600/3600))
        regen = 0;
        APP = 1;
        BPP = -b;
    elseif v == (25*(1600/3600))
        regen = 0.95;
        friction = 0.05;
        APP = 1 + b*regen;
        BPP = -b*friction;
    elseif v > (25*(1600/3600))
        regen = 0.95;
        friction = 0.05;
        APP = a + b*regen;
        BPP = -b*friction;
    else regen = (0.95/20)*v;
        friction = 1 - regen;
        APP = a + b*regen;
        BPP = -b*friction;
    end

    if SOC <= 0.1
        APP = 0;
        BPP = 0;
        regen = 0;
    end

== matlab function MEEN432_Project3_Wk3_Model/Throttle and Braking Logic/MATLAB Function1 ==
  data: regen input; vb output; v input
function vb = fcn(regen, v)

vb = regen*v;

== matlab function MEEN432_Project3_Wk3_Model/Long./Vehicle/MATLAB Function ==
  data: M input; acceleration output; Fw input; Fb input; Fd input; M_in input; Vy input; Omega input
function acceleration = fcn(M, Fw, Fb, Fd, M_in, Vy, Omega)

acceleration = ((Fw - Fb - Fd) / (M + M_in)) + Vy*Omega;

== matlab function MEEN432_Project3_Wk3_Model/SimpleLongVehicle/Tire Longitudinal Force/Tire Longitudinal Force ==
  data: lambda input; Fx output
function Fx = fcn(lambda)

y = u;

== matlab function MEEN432_Project3_Wk3_Model/Long./Wheel/MATLAB Function ==
  data: C0 input; Fdrag output; C1 input; C2 input; vel input
function Fdrag = fcn(C0, C1, C2, vel)

Fdrag = C0 + C1*vel + C2*vel^2;

== matlab function MEEN432_Project3_Wk3_Model/Long./Brake System/MATLAB Function ==
  data: alpha_b input; tau_b output; mu_b input; N_b_max input; g_b input; omega_w input
function tau_b = fcn(alpha_b, mu_b, N_b_max, g_b, omega_w)

N_b = alpha_b * N_b_max;
sgn = omega_w/(omega_w+0.0001);
tau_b = mu_b * N_b * g_b * sgn;

== matlab function MEEN432_Project3_Wk3_Model/SimpleLongVehicle/Tire Slip Ratio/Tire Slip Ratio ==
  data: v input; lambda output; r_w input; omega_w input
function lambda = fcn(v, r_w, omega_w)

if (r_w*omega_w - v) >= 0
    lambda = (r_w*omega_w - v)/(r_w*omega_w);
else
    lambda = (r_w*omega_w - v)/v;
end

== matlab function MEEN432_Project3_Wk3_Model/SimpleLongVehicle/Wheel Dynamics/Wheel Dynamics ==
  data: Fx input; omega_w_dot output; tau_w input; tau_b input; r_w input; I input
function omega_w_dot = fcn(Fx, tau_w, tau_b, r_w, I)

y = u;

== matlab function MEEN432_Project3_Wk3_Model/SimpleLongVehicle/Long Vehicle Dynamics/Long Vehicle Dynamics ==
  data: theta input; omega_dot output; Fx input; r input; F_drag input
function omega_dot = fcn(theta, Fx, r, F_drag)
g = 9.81;
omega_dot = (Fx*r - F_drag*r - m*g*r*sin(theta))/(m*r^2);

== matlab function MEEN432_Project3_Wk3_Model/SimpleLongVehicle/Braking/Braking ==
  data: alpha_b input; mu_b input; tau_b output; N_b_max input; g_b input; omega_w input
function tau_b = fcn(alpha_b, mu_b, N_b_max, g_b, omega_w)

N_b = alpha_b * N_b_max;

tau_b = mu_b * N_b * g_b * sign(omega_w);

== matlab function MEEN432_Project3_Wk3_Model/Throttle and Braking Logic/Driver (PID)/MATLAB Function ==
  data: v input; acc output; brake output
function [acc, brake] = fcn(v)

if v > 0
    acc = v;
    brake = 0;
elseif v < 0
    acc = 0;
    brake = v;
else
    acc = 0;
    brake = 0;
end

== matlab function MEEN432_Project3_Wk3_Model/SimpleLongVehiclewNoTireSlipAssumption1/MATLAB Function ==
  data: tau_w input; a output; tau_b input; r input; F_drag input; I_w input; m input
function a = fcn(tau_w, tau_b, r, F_drag, I_w, m)
theta = 90;
g = 9.81;

num = ((tau_w - tau_b) / r) - F_drag;
a = num / ((I_w / r^2) + m);

== matlab function MEEN432_Project3_Wk3_Model/Long./Electric Motor Drive/Electric Motor/MATLAB Function ==
  data: Tm input; I_bus output; Wm input; Effm input; V_bus input
function I_bus = fcn(Tm, Wm, Effm, V_bus)
    Pm = Tm*Wm;
    sgn_m = Pm / (abs(Pm) + 0.001);
    Pe = Pm / (Effm^sgn_m);
    if V_bus > 1
        I_bus = Pe/V_bus;
    else
        I_bus = 0;
    end

== matlab function MEEN432_Project3_Wk3_Model/Long./Electric Motor Drive/Inverter/MATLAB Function ==
  data: V_bat input; V_bus output; Eff_I input; I_bus input; I_bat output
function [V_bus, I_bat] = fcn(V_bat, Eff_I, I_bus)
    V_bus = V_bat; % Vbus = Vbat * r, where r is the inverter conversion ratio % * I_bat * Eff_I^(sgn_Pbat))/I_bus;
    P_bus = V_bus * I_bus;
    sgn_Pbus = P_bus / (abs(P_bus) + 0.001);

    if V_bus > 1
        I_bat = (P_bus / Eff_I^sgn_Pbus) / V_bat;
    else
        I_bat = 0;
    end
end

% double check ?
